simulink library "PredictionBlock"  (R2022a)
settings: Solver=VariableStepAuto  StartTime=0.0  StopTime=10.0  RelTol=1e-3
undefined symbols (not defined in the file): threshold
libraries: simulink x1, deeplib x1
settings Model: Creator=Alia  LastModifiedBy=Skander
settings SolverCC: AlgebraicLoopSolver=TrustRegion
settings DebuggingCC: UnconnectedInputMsg=warning  UnconnectedOutputMsg=warning  UnconnectedLineMsg=warning  SFMachineParentedDataDiag=warning
settings RTWCC: DLArmComputeVersion=19.05

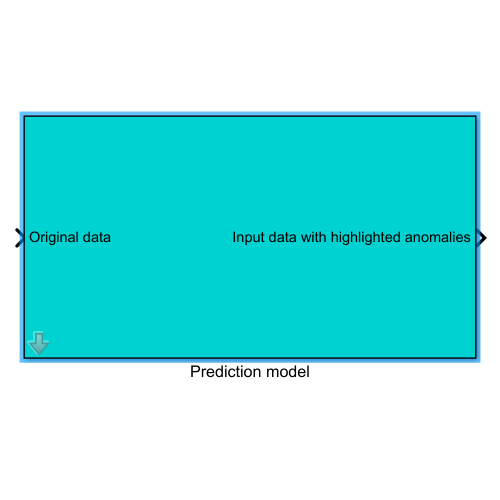
[thumbnail: Simulink's stored preview of the top-level diagram]
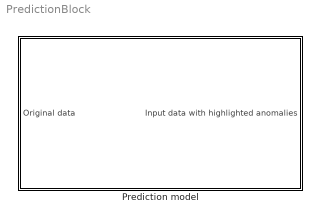
== system PredictionBlock ==
  Prediction model : Subsystem  mask{BufferLength=50, NetworkFilePath=C:\Users\Alia\Desktop\idriss\net.mat}
      mask prompts: BufferLength "dspshared:blkprm_prompts:OutputBufferSize"; NetworkFilePath "deep_blocks:common:FilePath"
      mask help: Buffer overload value must be equal to 1-BufferSize
      mask TypeOptions BufferLength:
      | Buffer timestamps /Buffer/N | Delay/DelayLength | Compare values to threshold/Compare
      | To Constant/const
      mask TypeOptions NetworkFilePath: Predictive network/NetworkFilePath
      mask DialogControl BufferLength Prompt: Output buffer size (per channel):
      mask DialogControl NetworkFilePath Prompt: File path:

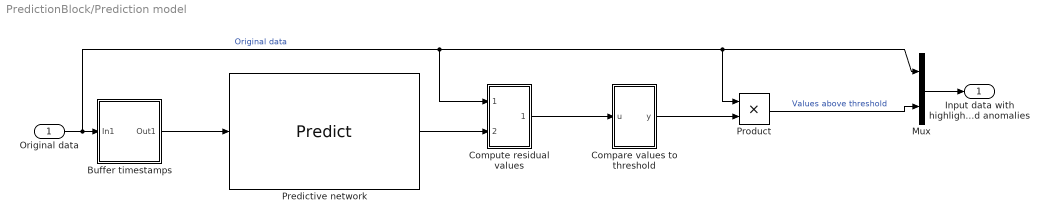
== system PredictionBlock/Prediction model ==
  Original data : Inport
  "Buffer timestamps " : Subsystem
  Compare values to threshold : Subsystem
  Compute residual values : Subsystem
  Mux : Mux  Inputs=2
  Predictive network : deeplib/Predict  Network=Network from MAT-file  NetworkFunction=squeezenet  NetworkFilePath=C:\Users\Alia\Desktop\idriss\net.mat  MiniBatchSize=128  InputDataFormats={ '', '' }  Predictions=on  Activations={}  ForceInterpretedSim=off  EnableDLNetwork=off
      settings: SourceProductBaseCode=NN
  Product : Product
  Input data with highlighted anomalies : Outport
  wires:
  Compute residual values/1(Out1) -> Compare values to threshold/1(u)
  Compare values to threshold/1(y) -> Product/2
  Original data/1 -> Product/1, Mux/1, Compute residual values/1(In1), "Buffer timestamps "/1(In1)  "Original data"
  Product/1 -> Mux/2  "Values above threshold"
  Mux/1 -> Input data with highlighted anomalies/1
  Predictive network/1 -> Compute residual values/2(In2)
  "Buffer timestamps "/1(Out1) -> Predictive network/1

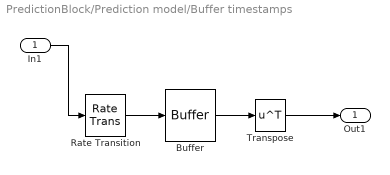
== system PredictionBlock/Prediction model/Buffer timestamps  ==
  In1 : Inport
  Buffer : Buffer  N=BufferLength  V=BufferLength-1  OutputFrames=off
  Rate Transition : RateTransition  OutPortSampleTime=1
  Transpose : Math  Operator=transpose
  Out1 : Outport
  wires:
  Rate Transition/1 -> Buffer/1
  Buffer/1 -> Transpose/1
  Transpose/1 -> Out1/1
  In1/1 -> Rate Transition/1

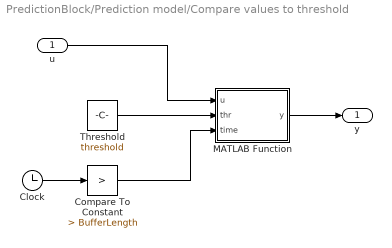
== system PredictionBlock/Prediction model/Compare values to threshold ==
  u : Inport
  Clock : Clock
  Compare To Constant : simulink/Logic and Bit Operations/Compare To Constant  relop=>  const=BufferLength  OutDataTypeStr=boolean
  MATLAB Function : MATLAB Function  TreatAsAtomicUnit=on
  Threshold : Constant  Value=threshold
  y : Outport
  wires:
  Compare To Constant/1 -> MATLAB Function/3(time)
  u/1 -> MATLAB Function/1(u)
  Clock/1 -> Compare To Constant/1
  Threshold/1 -> MATLAB Function/2(thr)
  MATLAB Function/1(y) -> y/1

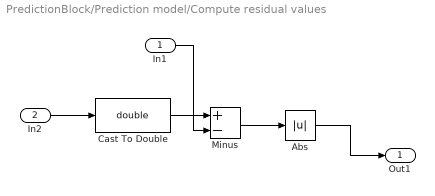
== system PredictionBlock/Prediction model/Compute residual values ==
  In1 : Inport
  In2 : Inport  Port=2
  Abs : Abs  SaturateOnIntegerOverflow=off
  Cast To Double : DataTypeConversion  OutDataTypeStr=double  SaturateOnIntegerOverflow=off  RndMeth=Floor
  Minus : Sum  Inputs=+-
  Out1 : Outport
  wires:
  Cast To Double/1 -> Minus/1
  In2/1 -> Cast To Double/1
  In1/1 -> Minus/2
  Abs/1 -> Out1/1
  Minus/1 -> Abs/1

== matlab function PredictionBlock/Prediction model/Compare values to threshold/MATLAB Function ==
  data: u input; y output; thr input; time input
function y = fcn(u,thr, time)
y = NaN;
if time == 1
    if u > thr
    y = 1;
    end
end
